simulink model "pidControllerAltitude"  (R2023b)
settings: Solver=VariableStepAuto  StartTime=0.0  StopTime=20  RelTol=1e-3
settings Model: Creator=mvhod  LastModifiedBy=mvhod

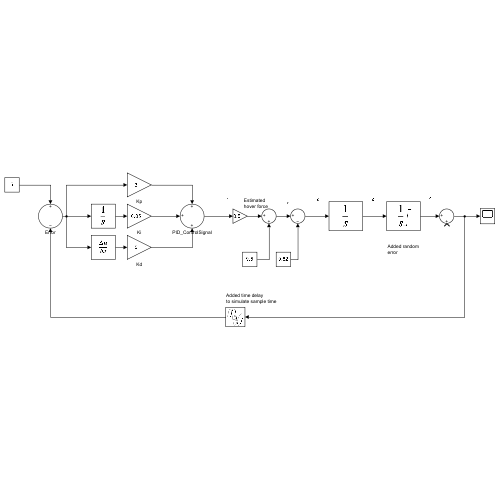
[thumbnail: Simulink's stored preview of the top-level diagram]
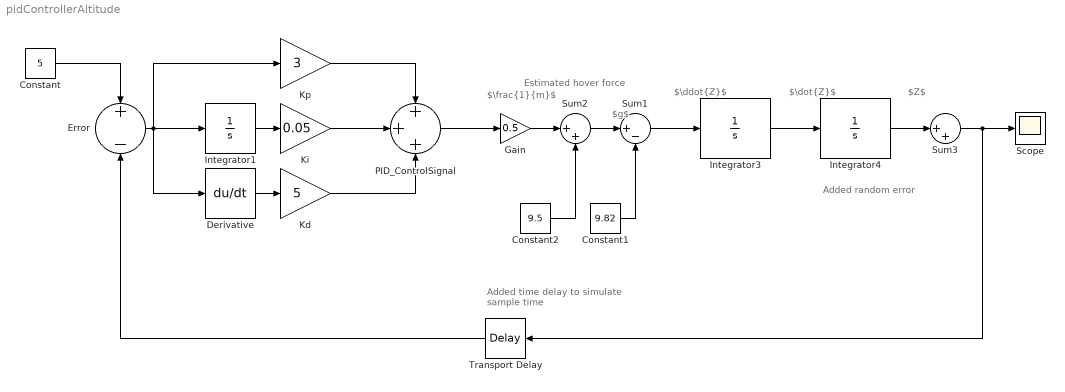
== system pidControllerAltitude ==
  note: $\ddot{Z}$
  note: Added random
      | error
  note: Estimated
      | hover force
  note: $\frac{1}{m}$
  note: $Z$
  note: Added time delay
      | to simulate sample time
  note: $g$
  note: $\dot{Z}$
  Constant : Constant  Value=5
  Constant1 : Constant  Value=9.82
  Constant2 : Constant  Value=9.5
  Derivative : Derivative
  Error : Sum  Inputs=+-
  Gain : Gain  Gain=0.5
  Integrator1 : Integrator
  Integrator3 : Integrator
  Integrator4 : Integrator  LimitOutput=on  LowerSaturationLimit=0
  Kd : Gain  Gain=5
  Ki : Gain  Gain=0.05
  Kp : Gain  Gain=3
  PID_ControlSignal : Sum  Inputs=+++
  Scope : Scope
  Sum1 : Sum  Inputs=|+-
  Sum2 : Sum  Inputs=|++
  Sum3 : Sum  Inputs=|++
  Transport Delay : TransportDelay  DelayTime=0.0000025
  wires:
  Integrator1/1 -> Ki/1
  Error/1 -> Integrator1/1, Derivative/1, Kp/1
  Derivative/1 -> Kd/1
  Kp/1 -> PID_ControlSignal/1
  Constant/1 -> Error/1
  PID_ControlSignal/1 -> Gain/1
  Ki/1 -> PID_ControlSignal/2
  Kd/1 -> PID_ControlSignal/3
  Sum3/1 -> Transport Delay/1, Scope/1
  Integrator3/1 -> Integrator4/1
  Constant2/1 -> Sum2/2
  Integrator4/1 -> Sum3/1
  Constant1/1 -> Sum1/2
  Gain/1 -> Sum2/1
  Sum2/1 -> Sum1/1
  Sum1/1 -> Integrator3/1
  Transport Delay/1 -> Error/2
